simulink model "SwitchRelay"  (R2025a)
settings: Solver=VariableStepAuto  StartTime=0.0  StopTime=10.0  RelTol=1e-3
settings Model: Creator=rivercovey  LastModifiedBy=rivercovey

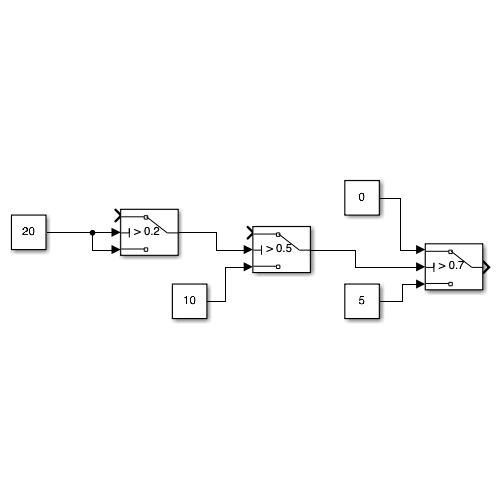
[thumbnail: Simulink's stored preview of the top-level diagram]
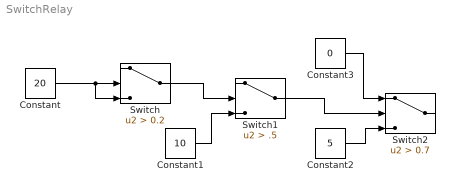
== system SwitchRelay ==
  Constant : Constant  Value=20
  Constant1 : Constant  Value=10
  Constant2 : Constant  Value=5
  Constant3 : Constant  Value=0
  Switch : Switch  Criteria=u2 > Threshold  Threshold=0.2  SaturateOnIntegerOverflow=off  InputSameDT=off
  Switch1 : Switch  Criteria=u2 > Threshold  Threshold=.5  SaturateOnIntegerOverflow=off  InputSameDT=off
  Switch2 : Switch  Criteria=u2 > Threshold  Threshold=0.7  SaturateOnIntegerOverflow=off  InputSameDT=off
  wires:
  Constant/1 -> Switch/3, Switch/2
  Switch/1 -> Switch1/2
  Constant1/1 -> Switch1/3
  Switch1/1 -> Switch2/2
  Constant3/1 -> Switch2/1
  Constant2/1 -> Switch2/3
